simulink model "project_new_automate_manual"  (R2020b)
settings: Solver=VariableStepAuto  StartTime=0.0  StopTime=inf  RelTol=1e-3
libraries: simulink x3
settings Model: EnablePacing=on  Creator=99003757  LastModifiedBy=99003757
settings ConfigComp: CovEnable=on  CovScope=ReferencedModels  CovIncludeTopModel=off  CovMetricSettings=dcmwe  CovModelRefEnable=on

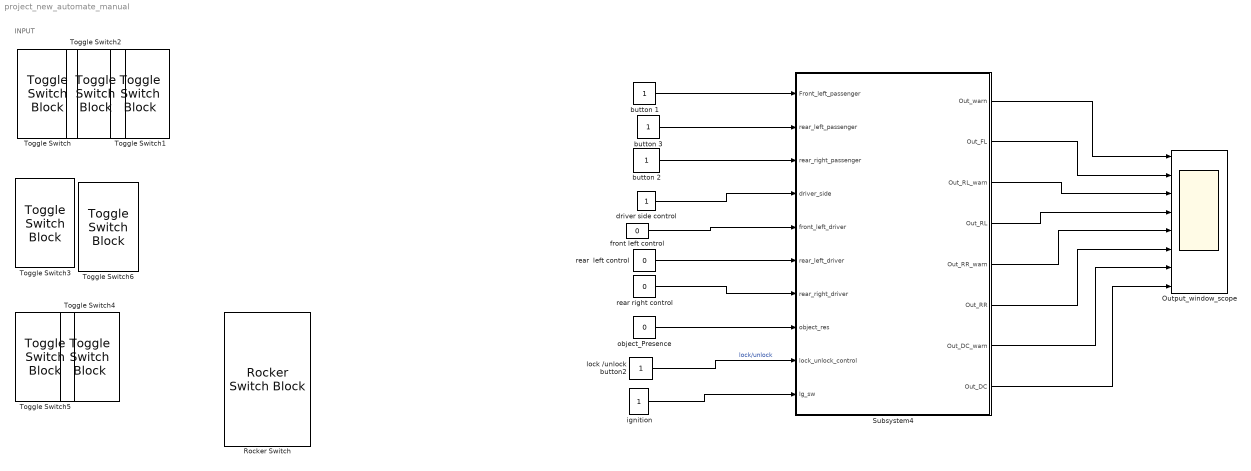
== system project_new_automate_manual ==
  note: INPUT
  Output_window_scope : Scope  NumInputPorts=8
  Rocker Switch : RockerSwitchBlock  LabelPosition=Bottom
      settings: Values={{'Off', 'On'}, [0 1]}
  Subsystem4 : Subsystem
  Toggle Switch{,1..6} (7 alike) : ToggleSwitchBlock
  "button 1 " : Constant
  button 2 : Constant
  button 3 : Constant
  driver side control : Constant
  front left control : Constant  Value=0
  "ignition " : Constant
  lock /unlock button2 : Constant
  object_Presence : Constant  Value=0
  rear  left control : Constant  Value=0
  rear right control : Constant  Value=0
  wires:
  Subsystem4/8(Out_DC) -> Output_window_scope/8
  Subsystem4/2(Out_FL) -> Output_window_scope/2
  Subsystem4/4(Out_RL) -> Output_window_scope/4
  Subsystem4/7(Out_DC_warn) -> Output_window_scope/7
  Subsystem4/6(Out_RR) -> Output_window_scope/6
  Subsystem4/5(Out_RR_warn) -> Output_window_scope/5
  Subsystem4/1(Out_warn) -> Output_window_scope/1
  Subsystem4/3(Out_RL_warn) -> Output_window_scope/3
  lock /unlock button2/1 -> Subsystem4/9(lock_unlock_control)  "lock/unlock"
  rear right control/1 -> Subsystem4/7(rear_right_driver)
  object_Presence/1 -> Subsystem4/8(object_res)
  rear  left control/1 -> Subsystem4/6(rear_left_driver)
  driver side control/1 -> Subsystem4/4(driver_side)
  front left control/1 -> Subsystem4/5(front_left_driver)
  "button 1 "/1 -> Subsystem4/1(Front_left_passenger)
  button 3/1 -> Subsystem4/2(rear_left_passenger)
  button 2/1 -> Subsystem4/3(rear_right_passenger)
  "ignition "/1 -> Subsystem4/10(Ig_sw)

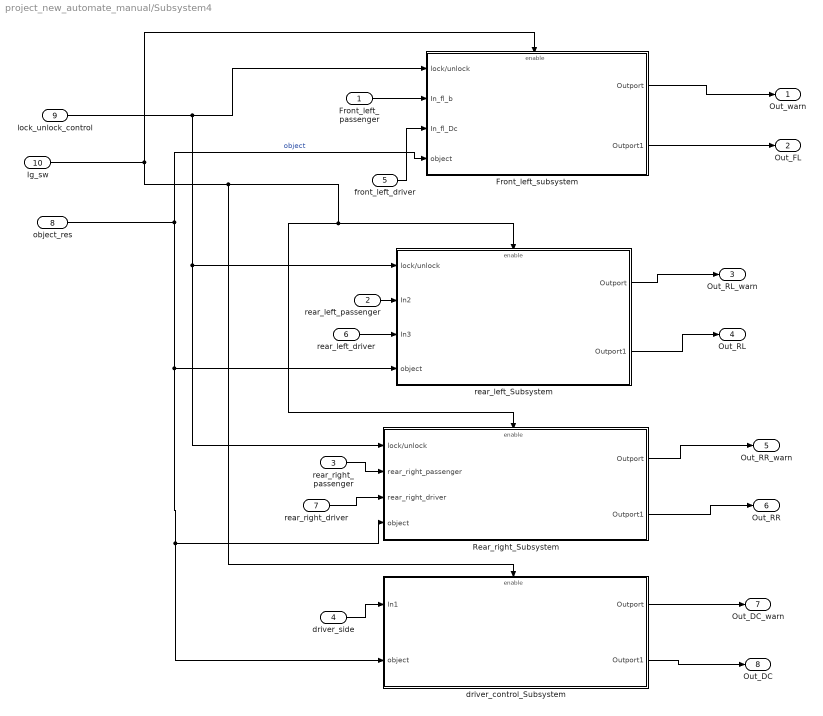
== system project_new_automate_manual/Subsystem4 ==
  Front_left_passenger : Inport
  rear_left_passenger : Inport  Port=2
  rear_right_passenger : Inport  Port=3
  driver_side : Inport  Port=4
  front_left_driver : Inport  Port=5
  rear_left_driver : Inport  Port=6
  rear_right_driver : Inport  Port=7
  object_res : Inport  Port=8
  lock_unlock_control : Inport  Port=9
  Ig_sw : Inport  Port=10
  Front_left_subsystem : Subsystem
  Rear_right_Subsystem : Subsystem
  driver_control_Subsystem : Subsystem
  rear_left_Subsystem : Subsystem
  Out_warn : Outport
  Out_FL : Outport  Port=2
  Out_RL_warn : Outport  Port=3
  Out_RL : Outport  Port=4
  Out_RR_warn : Outport  Port=5
  Out_RR : Outport  Port=6
  Out_DC_warn : Outport  Port=7
  Out_DC : Outport  Port=8
  wires:
  Ig_sw/1 -> Rear_right_Subsystem/Enable, rear_left_Subsystem/Enable, driver_control_Subsystem/Enable, Front_left_subsystem/Enable
  object_res/1 -> Front_left_subsystem/4(object), driver_control_Subsystem/2(object), Rear_right_Subsystem/4(object), rear_left_Subsystem/4(object)  "object"
  Front_left_subsystem/2(Outport1) -> Out_FL/1
  Front_left_subsystem/1(Outport) -> Out_warn/1
  rear_left_Subsystem/2(Outport1) -> Out_RL/1
  rear_left_Subsystem/1(Outport) -> Out_RL_warn/1
  Rear_right_Subsystem/2(Outport1) -> Out_RR/1
  Rear_right_Subsystem/1(Outport) -> Out_RR_warn/1
  driver_control_Subsystem/2(Outport1) -> Out_DC/1
  driver_control_Subsystem/1(Outport) -> Out_DC_warn/1
  Front_left_passenger/1 -> Front_left_subsystem/2(In_fl_b)
  front_left_driver/1 -> Front_left_subsystem/3(In_fl_Dc)
  rear_left_passenger/1 -> rear_left_Subsystem/2(In2)
  rear_left_driver/1 -> rear_left_Subsystem/3(In3)
  rear_right_passenger/1 -> Rear_right_Subsystem/2(rear_right_passenger)
  rear_right_driver/1 -> Rear_right_Subsystem/3(rear_right_driver)
  driver_side/1 -> driver_control_Subsystem/1(In1)
  lock_unlock_control/1 -> Rear_right_Subsystem/1(lock/unlock), rear_left_Subsystem/1(lock/unlock), Front_left_subsystem/1(lock/unlock)

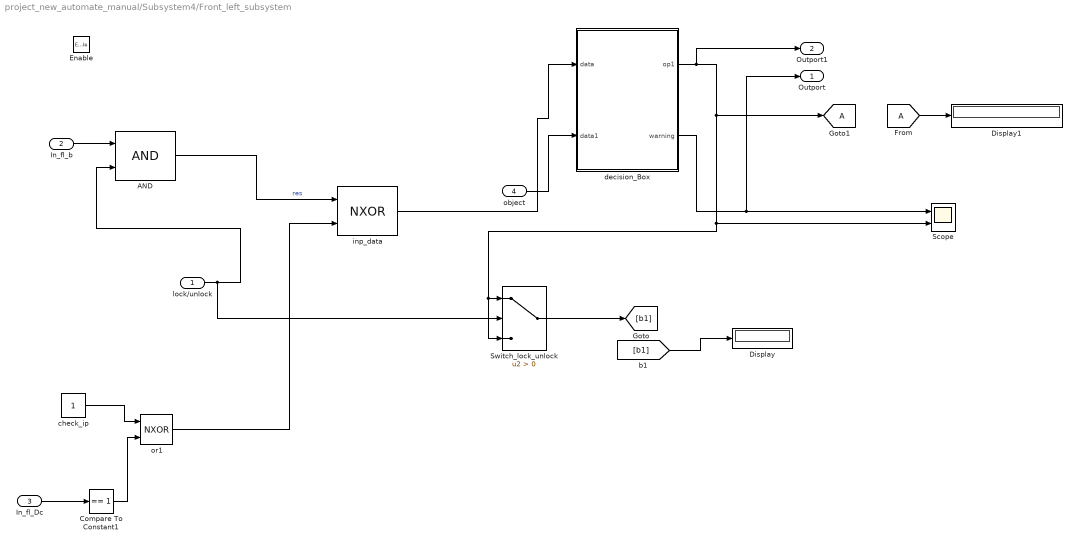
== system project_new_automate_manual/Subsystem4/Front_left_subsystem ==
  lock/unlock : Inport
  In_fl_b : Inport  Port=2
  In_fl_Dc : Inport  Port=3
  object : Inport  Port=4
  Enable : EnablePort
  AND : Logic  IconShape=distinctive  AllPortsSameDT=off  OutDataTypeStr=boolean
  Compare To Constant1 : simulink/Logic and Bit Operations/Compare To Constant  relop===  const=1  OutDataTypeStr=boolean
  Display : Display
  Display1 : Display
  Scope : Scope  NumInputPorts=2
  Switch_lock_unlock : Switch  Criteria=u2 > Threshold
  check_ip : Constant
  decision_Box : Stateflow chart  TreatAsAtomicUnit=on
  inp_data : Logic  Operator=NXOR  IconShape=distinctive  AllPortsSameDT=off  OutDataTypeStr=boolean
  or1 : Logic  Operator=NXOR  IconShape=distinctive  AllPortsSameDT=off  OutDataTypeStr=boolean
  Outport : Outport
  Outport1 : Outport  Port=2
  tag scope: A=global
  wires:
  In_fl_b/1 -> AND/1
  check_ip/1 -> or1/1
  Switch_lock_unlock/1 -> [b1]
  Compare To Constant1/1 -> or1/2
  [b1] -> Display/1
  decision_Box/1(op1) -> Outport1/1, Switch_lock_unlock/3, Switch_lock_unlock/1, Scope/2, [A]
  decision_Box/2(warning) -> Outport/1, Scope/1
  object/1 -> decision_Box/2(data1)
  [A] -> Display1/1
  inp_data/1 -> decision_Box/1(data)
  In_fl_Dc/1 -> Compare To Constant1/1
  AND/1 -> inp_data/1  "res"
  or1/1 -> inp_data/2
  lock/unlock/1 -> Switch_lock_unlock/2, AND/2

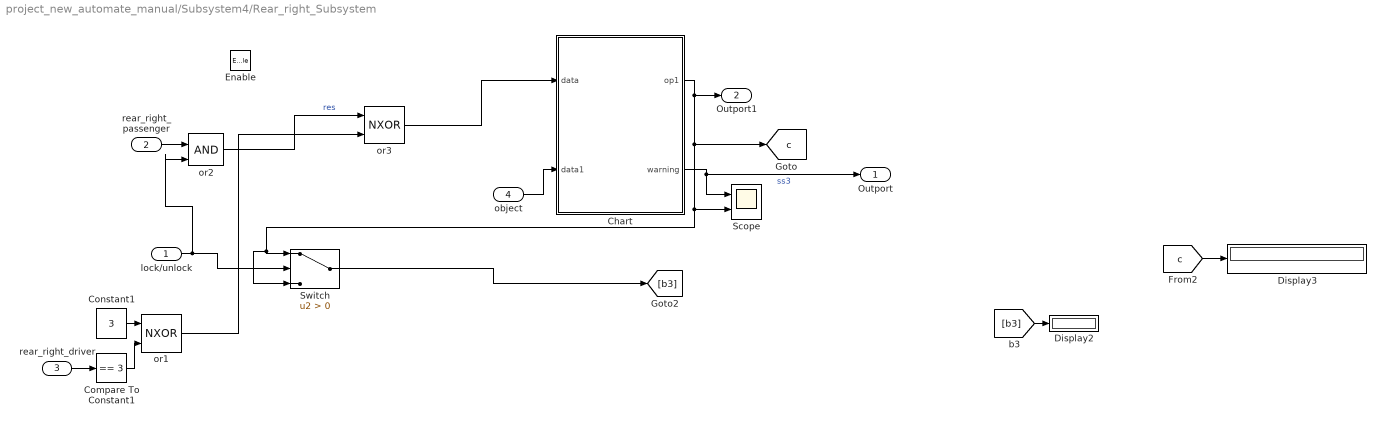
== system project_new_automate_manual/Subsystem4/Rear_right_Subsystem ==
  lock/unlock : Inport
  rear_right_passenger : Inport  Port=2
  rear_right_driver : Inport  Port=3
  object : Inport  Port=4
  Enable : EnablePort
  Chart : Stateflow chart  TreatAsAtomicUnit=on
  Compare To Constant1 : simulink/Logic and Bit Operations/Compare To Constant  relop===  const=3  OutDataTypeStr=boolean
  Constant1 : Constant  Value=3
  Display2 : Display
  Display3 : Display
  Scope : Scope  NumInputPorts=2
  Switch : Switch  Criteria=u2 > Threshold
  or1 : Logic  Operator=NXOR  IconShape=distinctive  AllPortsSameDT=off  OutDataTypeStr=boolean
  or2 : Logic  IconShape=distinctive  AllPortsSameDT=off  OutDataTypeStr=boolean
  or3 : Logic  Operator=NXOR  IconShape=distinctive  AllPortsSameDT=off  OutDataTypeStr=boolean
  Outport : Outport
  Outport1 : Outport  Port=2
  tag scope: c=global
  wires:
  Constant1/1 -> or1/1
  [b3] -> Display2/1
  Compare To Constant1/1 -> or1/2
  Switch/1 -> [b3]
  lock/unlock/1 -> or2/2, Switch/2
  Chart/2(warning) -> Scope/1, Outport/1  "ss3"
  object/1 -> Chart/2(data1)
  or1/1 -> or3/2
  or2/1 -> or3/1  "res"
  or3/1 -> Chart/1(data)
  [c] -> Display3/1
  Chart/1(op1) -> Outport1/1, [c], Scope/2, Switch/3, Switch/1
  rear_right_passenger/1 -> or2/1
  rear_right_driver/1 -> Compare To Constant1/1

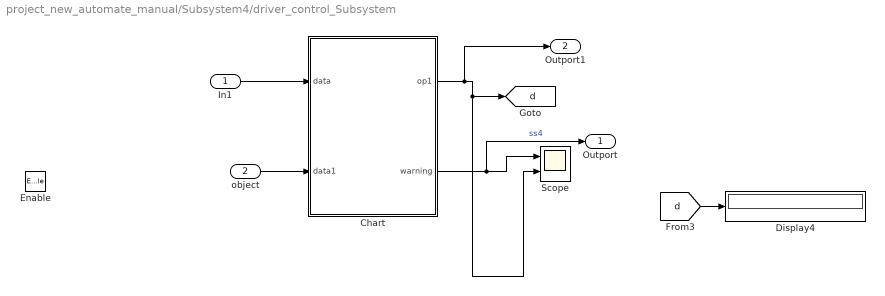
== system project_new_automate_manual/Subsystem4/driver_control_Subsystem ==
  In1 : Inport
  object : Inport  Port=2
  Enable : EnablePort
  Chart : Stateflow chart  TreatAsAtomicUnit=on
  Display4 : Display
  Scope : Scope  NumInputPorts=2
  Outport : Outport
  Outport1 : Outport  Port=2
  tag scope: d=global
  wires:
  Chart/2(warning) -> Outport/1, Scope/1  "ss4"
  object/1 -> Chart/2(data1)
  In1/1 -> Chart/1(data)
  [d] -> Display4/1
  Chart/1(op1) -> Outport1/1, [d], Scope/2

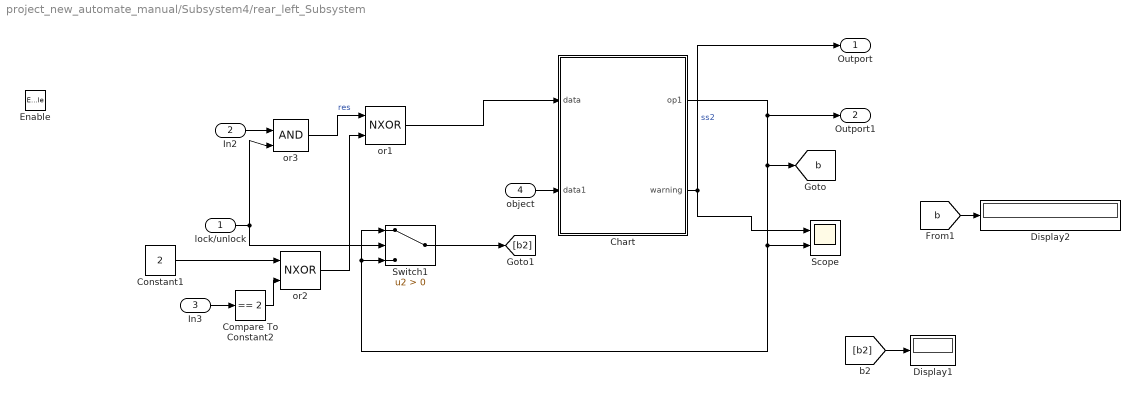
== system project_new_automate_manual/Subsystem4/rear_left_Subsystem ==
  lock/unlock : Inport
  In2 : Inport  Port=2
  In3 : Inport  Port=3
  object : Inport  Port=4
  Enable : EnablePort
  Chart : Stateflow chart  TreatAsAtomicUnit=on
  Compare To Constant2 : simulink/Logic and Bit Operations/Compare To Constant  relop===  const=2  OutDataTypeStr=boolean
  Constant1 : Constant  Value=2
  Display1 : Display
  Display2 : Display
  Scope : Scope  NumInputPorts=2
  Switch1 : Switch  Criteria=u2 > Threshold
  or1 : Logic  Operator=NXOR  IconShape=distinctive  AllPortsSameDT=off  OutDataTypeStr=boolean
  or2 : Logic  Operator=NXOR  IconShape=distinctive  AllPortsSameDT=off  OutDataTypeStr=boolean
  or3 : Logic  IconShape=distinctive  AllPortsSameDT=off  OutDataTypeStr=boolean
  Outport : Outport
  Outport1 : Outport  Port=2
  tag scope: b=global
  wires:
  [b2] -> Display1/1
  Constant1/1 -> or2/1
  Compare To Constant2/1 -> or2/2
  Switch1/1 -> [b2]
  lock/unlock/1 -> Switch1/2, or3/2
  object/1 -> Chart/2(data1)
  Chart/2(warning) -> Outport/1, Scope/1  "ss2"
  or3/1 -> or1/1  "res"
  or2/1 -> or1/2
  or1/1 -> Chart/1(data)
  [b] -> Display2/1
  Chart/1(op1) -> Outport1/1, [b], Switch1/3, Switch1/1, Scope/2
  In2/1 -> or3/1
  In3/1 -> Compare To Constant2/1

== stateflow chart project_new_automate_manual/Subsystem4/Front_left_subsystem/decision_Box ==
  state Normal
    state Start
      entry:
      op1 = 25;
    state second
      entry:
      op1 = 100;
    state PrepareToStop
      entry:
      op1 = 75;
    state Go
      % Green light
      entry:
      op1 = 50;
    (default) -> Start
    Start -> (junction 9)
    (junction 9) -> (junction 6) : after(1,sec)
    PrepareToStop -> second : after(1,sec)
    (junction 6) -> Go
    Go -> PrepareToStop : after(1,sec)
  state Fault
    entry:
    op1 =0;
    state BlinkOn
      % Red light
      entry:
      warning = 1;
    (default) -> BlinkOn
  state block_start
    entry:
  state Normal2
    state state5
      entry:
      op1=0
    state Start1
      entry:
      op1=op1;
    state two
      entry:
      op1 = 0;
    state four3
      entry:
      op1 = 0;
    state three
      entry:
      op1 = 25;
    state three1
      entry:
      op1 = 0;
    state five2
      entry:
      op1=0;
    state five
      entry:
      op1=50;
    state five1
      entry:
      op1=25;
    state four2
      entry:
      op1 = 25;
    state four
      entry:
      op1 = 75;
    state four1
      entry:
      op1 = 50;
    Start1 -> state5 [order 4] : [op1==0]
    (default) -> Start1
    Start1 -> (junction 143) [order 2] : after(1,sec)[op1==25]
    (junction 143) -> four3
    Start1 -> (junction 89) [order 3]
    Start1 -> (junction 103) [order 5]
    Start1 -> (junction 48) [order 1]
    (junction 103) -> (junction 104) : after(1,sec)[op1==50]
    (junction 48) -> (junction 49) : after(1,sec)[op1==100]
    (junction 89) -> (junction 90) : after(1,sec)[op1==75]
    three -> two : after(1,sec)[op1==25]
    (junction 104) -> four2
    (junction 49) -> four
    five -> three : after(1,sec)[op1==50]
    (junction 90) -> four1
    five1 -> three1 : after(1,sec)[op1==25]
    four2 -> five2 : after(1,sec)[op1==25]
    four -> five : after(1,sec)[op1==75]
    four1 -> five1 : after(1,sec)[op1==50]
  (default) -> block_start
  block_start -> Normal2 [order 2] : [data == 0]
  Normal -> Fault [order 1] : [data1 == 1]
  block_start -> Normal [order 1] : [data ==1 ]
  Normal2 -> block_start [order 1] : [data ==1]
  Normal -> block_start [order 2] : [data == 0]
  Fault -> Normal [order 1] : [data1 == 0]
  Fault -> Normal2 [order 2] : [data1 ==0]
  Normal2 -> Fault [order 2] : [data1==1]
  data: data input; data1 input; op1 output =0; warning output

== stateflow chart project_new_automate_manual/Subsystem4/Rear_right_Subsystem/Chart ==
  state Normal
    state Start
      entry:
      op1 = 25;
    state second
      entry:
      op1 = 100;
    state PrepareToStop
      entry:
      op1 = 75;
    state Go
      % Green light
      entry:
      op1 = 50;
    (default) -> Start
    Start -> (junction 9)
    (junction 9) -> (junction 6) : after(1,sec)
    PrepareToStop -> second : after(1,sec)
    (junction 6) -> Go
    Go -> PrepareToStop : after(1,sec)
  state Fault
    entry:
    op1 =0;
    state BlinkOn
      % Red light
      entry:
      warning = 1;
    (default) -> BlinkOn
  state block_start
    entry:
  state Normal2
    state state5
      entry:
      op1=0
    state Start1
      entry:
    state two
      entry:
      op1 = 0;
    state four3
      entry:
      op1 = 0;
    state three
      entry:
      op1 = 25;
    state three1
      entry:
      op1 = 0;
    state five2
      entry:
      op1=0;
    state five
      entry:
      op1=50;
    state five1
      entry:
      op1=25;
    state four2
      entry:
      op1 = 25;
    state four
      entry:
      op1 = 75;
    state four1
      entry:
      op1 = 50;
    Start1 -> state5 [order 2] : [op1==0]
    (default) -> Start1
    Start1 -> (junction 143) [order 3] : after(1,sec)[op1==25]
    (junction 143) -> four3
    Start1 -> (junction 89) [order 4]
    Start1 -> (junction 103) [order 5]
    Start1 -> (junction 48) [order 1]
    (junction 103) -> (junction 104) : after(1,sec)[op1==50]
    (junction 48) -> (junction 49) : after(1,sec)[op1==100]
    (junction 89) -> (junction 90) : after(1,sec)[op1==75]
    three -> two : after(1,sec)[op1==25]
    (junction 104) -> four2
    (junction 49) -> four
    five -> three : after(1,sec)[op1==50]
    (junction 90) -> four1
    five1 -> three1 : after(1,sec)[op1==25]
    four2 -> five2 : after(1,sec)[op1==25]
    four -> five : after(1,sec)[op1==75]
    four1 -> five1 : after(1,sec)[op1==50]
  (default) -> block_start
  block_start -> Normal2 [order 2] : [data == 0]
  Normal -> Fault [order 1] : [data1 == 1]
  block_start -> Normal [order 1] : [data ==1]
  Normal2 -> block_start [order 1] : [data ==1]
  Normal -> block_start [order 2] : [data ==0]
  Fault -> Normal [order 1] : [data1 == 0]
  Fault -> Normal2 [order 2] : [data1 ==0]
  Normal2 -> Fault [order 2] : [data1==1]
  data: data input; data1 input; op1 output =0; warning output

== stateflow chart project_new_automate_manual/Subsystem4/driver_control_Subsystem/Chart ==
  state Normal
    state Start
      entry:
      op1 = 25;
    state second
      entry:
      op1 = 100;
    state PrepareToStop
      entry:
      op1 = 75;
    state Go
      % Green light
      entry:
      op1 = 50;
    (default) -> Start
    Start -> (junction 9)
    (junction 9) -> (junction 6) : after(1,sec)
    PrepareToStop -> second : after(1,sec)
    (junction 6) -> Go
    Go -> PrepareToStop : after(1,sec)
  state Fault
    entry:
    op1 =0;
    state BlinkOn
      % Red light
      entry:
      warning = 1;
    (default) -> BlinkOn
  state block_start
    entry:
  state Normal2
    state state5
      entry:
      op1=0
    state Start1
      entry:
      op1=op1;
    state two
      entry:
      op1 = 0;
    state four3
      entry:
      op1 = 0;
    state three
      entry:
      op1 = 25;
    state three1
      entry:
      op1 = 0;
    state five2
      entry:
      op1=0;
    state five
      entry:
      op1=50;
    state five1
      entry:
      op1=25;
    state four2
      entry:
      op1 = 25;
    state four
      entry:
      op1 = 75;
    state four1
      entry:
      op1 = 50;
    Start1 -> state5 [order 4] : [op1==0]
    (default) -> Start1
    Start1 -> (junction 142) [order 2] : after(1,sec)[op1==25]
    Start1 -> (junction 89) [order 3]
    Start1 -> (junction 103) [order 5]
    (junction 142) -> four3
    Start1 -> (junction 48) [order 1]
    (junction 103) -> (junction 104) : after(1,sec)[op1==50]
    (junction 48) -> (junction 49) : after(1,sec)[op1==100]
    (junction 89) -> (junction 90) : after(1,sec)[op1==75]
    three -> two : after(1,sec)[op1==25]
    (junction 104) -> four2
    (junction 49) -> four
    five -> three : after(1,sec)[op1==50]
    (junction 90) -> four1
    five1 -> three1 : after(1,sec)[op1==25]
    four2 -> five2 : after(1,sec)[op1==25]
    four -> five : after(1,sec)[op1==75]
    four1 -> five1 : after(1,sec)[op1==50]
  (default) -> block_start
  block_start -> Normal2 [order 2] : [data == 0]
  Normal -> Fault [order 1] : [data1 == 1]
  block_start -> Normal [order 1] : [data ==1]
  Normal2 -> block_start [order 1] : [data ==1]
  Normal -> block_start [order 2] : [data ==0]
  Fault -> Normal [order 1] : [data1 == 0]
  Fault -> Normal2 [order 2] : [data1 ==0]
  Normal2 -> Fault [order 2] : [data1==1]
  data: data input; data1 input; op1 output =0; warning output

== stateflow chart project_new_automate_manual/Subsystem4/rear_left_Subsystem/Chart ==
  state Normal
    state Start
      entry:
      op1 = 25;
    state second
      entry:
      op1 = 100;
    state PrepareToStop
      entry:
      op1 = 75;
    state Go
      % Green light
      entry:
      op1 = 50;
    (default) -> Start
    Start -> (junction 9)
    (junction 9) -> (junction 6) : after(1,sec)
    PrepareToStop -> second : after(1,sec)
    (junction 6) -> Go
    Go -> PrepareToStop : after(1,sec)
  state Fault
    entry:
    op1 =0;
    state BlinkOn
      % Red light
      entry:
      warning = 1;
    (default) -> BlinkOn
  state block_start
    entry:
  state Normal2
    state state5
      entry:
      op1=0
    state Start1
      entry:
      op1=op1;
    state two
      entry:
      op1 = 0;
    state four3
      entry:
      op1 = 0;
    state three
      entry:
      op1 = 25;
    state three1
      entry:
      op1 = 0;
    state five2
      entry:
      op1=0;
    state five
      entry:
      op1=50;
    state five1
      entry:
      op1=25;
    state four2
      entry:
      op1 = 25;
    state four
      entry:
      op1 = 75;
    state four1
      entry:
      op1 = 50;
    Start1 -> state5 [order 4] : [op1==0]
    (default) -> Start1
    Start1 -> (junction 142) [order 2] : after(1,sec)[op1==25]
    (junction 142) -> four3
    Start1 -> (junction 89) [order 3]
    Start1 -> (junction 103) [order 5]
    Start1 -> (junction 48) [order 1]
    (junction 103) -> (junction 104) : after(1,sec)[op1==50]
    (junction 48) -> (junction 49) : after(1,sec)[op1==100]
    (junction 89) -> (junction 90) : after(1,sec)[op1==75]
    three -> two : after(1,sec)[op1==25]
    (junction 104) -> four2
    (junction 49) -> four
    five -> three : after(1,sec)[op1==50]
    (junction 90) -> four1
    five1 -> three1 : after(1,sec)[op1==25]
    four2 -> five2 : after(1,sec)[op1==25]
    four -> five : after(1,sec)[op1==75]
    four1 -> five1 : after(1,sec)[op1==50]
  (default) -> block_start
  block_start -> Normal2 [order 2] : [data == 0]
  Normal -> Fault [order 1] : [data1 == 1]
  block_start -> Normal [order 1] : [data ==1]
  Normal2 -> block_start [order 1] : [data ==1]
  Normal -> block_start [order 2] : [data ==0]
  Fault -> Normal [order 1] : [data1 == 0]
  Fault -> Normal2 [order 2] : [data1 ==0]
  Normal2 -> Fault [order 2] : [data1==1]
  data: data input; data1 input; op1 output =0; warning output
